simulink model "Wind_Turbine_Model"  (R2023a)
settings: Solver=VariableStepAuto  StartTime=0.0  StopTime=65  RelTol=1e-3
values from neighbouring files (symbols this model uses):
  Cbus = 80e-3*n_wt_agg*u^2    (= 1.33333333333)    [param.m]
  D = 1e-3    (= 0.001)    [param.m]
  f = 50    [param.m]
  Fs = Vs * sqrt(2/3)/(2*pi*f)    [param.m]
  fsw = 4e3    (= 4000)    [param.m]
  Idr_rated = sqrt(2)*Is    [param.m]
  J = 127*n_wt_agg    (= 19050)    [param.m]
  ki_id = (wni^2)*Lr*sigma    (= 3.27733001332)    [param.m]
  ki_idg = (wnig^2)*Lg    (= 0.263189450696)    [param.m]
  ki_iq = ki_id    (= 3.27733001332)    [param.m]
  ki_iqg = ki_idg    (= 0.263189450696)    [param.m]
  ki_v = -300000*n_wt_agg    (= -45000000)    [param.m]
  Kopt = ((0.5*rho*pi*(Radius^5)*Cp_max)/(lambda_opt^3))    (= 296454.198186)    [param.m]
  kp_id = (2*wni*sigma*Lr) - Rr    (= 0.00384733333333)    [param.m]
  kp_idg = ((2*wnig*Lg)-Rg)    (= 0.00167538274858)    [param.m]
  kp_iq = kp_id    (= 0.00384733333333)    [param.m]
  kp_iqg = kp_idg    (= 0.00167538274858)    [param.m]
  kp_v = -1000*n_wt_agg    (= -150000)    [param.m]
  Kpg = 1/(1.5*Vr*sqrt(2/3))    [param.m]
  Kqg = -Kpg    [param.m]
  lambda_opt = 7.2    [param.m]
  Lg = 400e-6 /n_wt_agg    (= 2.66666666667e-06)    [param.m]
  Lm = 2.5e-3 /n_wt_agg    (= 1.66666666667e-05)    [param.m]
  Lr = Lm + Lsi    (= 1.72466666667e-05)    [param.m]
  Ls = Lm + Lsi    (= 1.72466666667e-05)    [param.m]
  Lsi = 0.087e-3 /n_wt_agg    (= 5.8e-07)    [param.m]
  N = 100    [param.m]
  n_wt_agg = 150    [param.m]
  p = 2    [param.m]
  Ps = 2e6*n_wt_agg    (= 300000000)    [param.m]
  Radius = 42    [param.m]
  Rg = 20e-6 /n_wt_agg    (= 1.33333333333e-07)    [param.m]
  rho = 1.225    [param.m]
  Rr = 2.9e-3 /n_wt_agg    (= 1.93333333333e-05)    [param.m]
  Rs = 2.6e-3 /n_wt_agg    (= 1.73333333333e-05)    [param.m]
  sigma = 1 - Lm^2 / (Ls*Lr)    (= 0.0661284179513)    [param.m]
  smax = 1/3    (= 0.333333333333)    [param.m]
  tab_lambda = [0.1:0.01:11.8]    [param.m]
  Ts = 1/fsw/50    (= 5e-06)    [param.m]
  Vbus = 1150/u    (= 3450)    [param.m]
  Vs = 690    [param.m]
undefined symbols (not defined in the file or in its folder): Cp, DiscIntNeverNeededParam
libraries: spsSecondOrderFilterLib x10, simulink x5, spsThreePhaseVIMeasurementLib x4, spsPower3phInstantaneousLib x4, spsPiSectionLineLib x3, spsGroundLib x3, spsThreePhaseTransformerTwoWindingsLib x2, spsThreePhaseProgrammableVoltageSourceLib x2, spsUniversalBridgeLib x2, spsPWMGenerator2LevelLib x2, spsThreePhaseSeriesRLCBranchLib x2, spsAsynchronousMachineSIUnitsLib x1
(part 1 of 2)
settings Model: Creator=deleersnijde  LastModifiedBy=gdemuyter
settings DataIOCC: ReturnWorkspaceOutputs=off
settings RTWCC: GPUComputeCapability=5.0

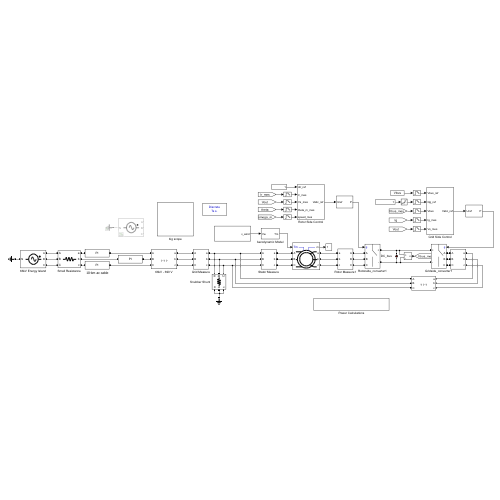
[thumbnail: Simulink's stored preview of the top-level diagram]
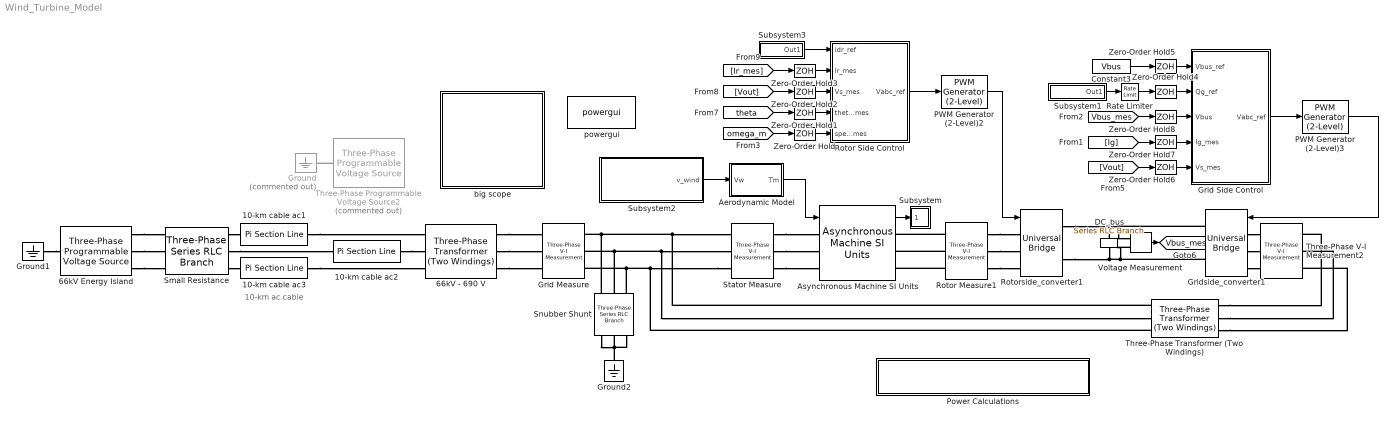
== system Wind_Turbine_Model ==
  note: 10-km ac cable
  10-km cable ac1 : spsPiSectionLineLib/Pi Section Line  LConnTagsString=__new0  RConnTagsString=__new0  Phases=1  PiSections=2  Length=10  Frequency=50  Resistance=0.034/(n_wt_agg/35)  Inductance=0.34e-3/(n_wt_agg/35)  Capacitance=0.29e-06*(n_wt_agg/35)  SpecifyConductance=off  Conductance=0  Measurements=None  Measurements2=None
  10-km cable ac2 : spsPiSectionLineLib/Pi Section Line  LConnTagsString=__new0  RConnTagsString=__new0  Phases=1  PiSections=2  Length=10  Frequency=50  Resistance=0.034/(n_wt_agg/35)  Inductance=0.34e-3/(n_wt_agg/35)  Capacitance=0.29e-06*(n_wt_agg/35)  SpecifyConductance=off  Conductance=0  Measurements=None  Measurements2=None
  10-km cable ac3 : spsPiSectionLineLib/Pi Section Line  LConnTagsString=__new0  RConnTagsString=__new0  Phases=1  PiSections=2  Length=10  Frequency=50  Resistance=0.034/(n_wt_agg/35)  Inductance=0.34e-3/(n_wt_agg/35)  Capacitance=0.29e-06*(n_wt_agg/35)  SpecifyConductance=off  Conductance=0  Measurements=None  Measurements2=None
  66kV - 690 V : spsThreePhaseTransformerTwoWindingsLib/Three-Phase Transformer (Two Windings)  Winding1Connection=Yg  Winding2Connection=Yg  CoreType=Three single-phase transformers  SetSaturation=off  Hysteresis=off  DataFile='hysteresis'  SetInitialFlux=off  Measurements=None  UNITS=pu  NominalPower=[ Ps , f ]  Winding1=[66000 0.025/100/25 0.015/25]  Winding2=[Vs 0.025/100/25 0.015/25]  Rm=500  Lm=500  L0=0.5  Saturation=[0 0;0.22957 0.012546;95.654 0.015891]  InitialFluxes=[ 0.8 , -0.8 , 0.7 ]  BreakLoop=off  DiscreteSolver=Trapezoidal iterative  DataType=off  TransfoNumber=1
  66kV Energy Island : spsThreePhaseProgrammableVoltageSourceLib/Three-Phase Programmable Voltage Source  PositiveSequence=[66e3 0 f]  VariationEntity=Amplitude  VariationType=Table of time-amplitude pairs  VariationTypeAlt=Step  VariationStep=0.5  VariationRate=10  VariationMagnitude=0.3  VariationFrequency=2  VariationTiming=[1 2]  VariationPhaseA=off  Amplitudes=[1 0.8 0.9 1.0]  TimeValues=[0 45 45.3 50]  HarmonicGeneration=off  HarmonicA=[3 0.2 -25 0]  HarmonicB=[2 0.15 35 2]  Timing="[0.05  3]"  BusType=swing  Pref=0  Qref=0  Qmin=-inf  Qmax=inf
  Aerodynamic Model : Subsystem
  Asynchronous Machine SI Units : spsAsynchronousMachineSIUnitsLib/Asynchronous Machine SI Units  RotorType=Wound  PresetModel=No  MechanicalLoad=Torque Tm  ShowDetailedParameters=on  ReferenceFrame=Rotor  Units=SI  MeasurementBus=off  NominalParameters=[Ps Vs f]  VoltageRatio=1/u  Stator=[Rs Lsi]  Rotor=[Rr Lsi]  Cage1=[0.4155 0.002066]  Cage2=[0.4168 0.0003495]  Lm=Lm  Mechanical=[J D 2]  PolePairs=2  InitialConditions=[0.454 0 0 0 0 0 0 0]  SimulateSaturation=off  Saturation=[14.03593122, 27.81365428, 53.79336849, 72.68890987, 97.98006896, 148.6815601, 215.7428561, 302.9841135, 428.7778367 ; 230, 322, 414, 460, 506, 552, 598, 644, 690]  LoadFlowParameters=1492000  TsPowergui=0  TsBlock=-1  IterativeModel=Trapezoidal non iterative  IterativeDiscreteModel=Trapezoidal non iterative  Pmec=1.492e+006
  Constant3 : Constant  Value=Vbus
  DC_bus : spsSeriesRLCBranchLib/Series RLC Branch  LConnTagsString=__new0  RConnTagsString=__new0  BranchType=C  Resistance=1  Inductance=1e-3  SetiL0=off  InitialCurrent=0  Capacitance=Cbus  Setx0=on  InitialVoltage=Vbus  Measurements=Branch voltage
  Grid Measure : spsThreePhaseVIMeasurementLib/Three-Phase V-I Measurement  VoltageMeasurement=phase-to-ground  SetLabelV=on  LabelV=Vout  Vpu=off  VpuLL=off  CurrentMeasurement=yes  SetLabelI=on  LabelI=Iout  Ipu=off  Pbase=100e6  Vbase=500e3  OutputType=Complex  PhasorSimulation=off  PSBequivalent=0
  Grid Side Control : Subsystem
  Gridside_converter1 : spsUniversalBridgeLib/Universal Bridge  Arms=3  SnubberResistance=5000  SnubberCapacitance=1e-6  Device=Ideal Switches  Ron=1e-3  Lon=0  ForwardVoltages="[  0  0  ]"  ForwardVoltage=0  GTOparameters=[ 10e-6 , 20e-6 ]  IGBTparameters=[ 1e-6 , 2e-6 ]  Measurements=UAB UBC UCA UDC voltages  Measurements_2=None  converterType=Rectifier
  Ground : spsGroundLib/Ground  Commented=on  LConnTagsString=a
  Ground1 : spsGroundLib/Ground  LConnTagsString=a
  Ground2 : spsGroundLib/Ground  LConnTagsString=a
  PWM Generator (2-Level)2 : spsPWMGenerator2LevelLib/PWM Generator (2-Level)  ModulatorType=Three-phase bridge (6 pulses)  ModulatorMode=Unsynchronized  Fc=fsw  Pc=0  nF=27  MinMax="[ -1  1 ]"  SamplingTechnique=Symmetrical regular (single edge)  ModulatingSignals=off  m=0.8  Freq=60  Phase=0  Ts=0  ShowCarrierOutport=off
  PWM Generator (2-Level)3 : spsPWMGenerator2LevelLib/PWM Generator (2-Level)  ModulatorType=Three-phase bridge (6 pulses)  ModulatorMode=Unsynchronized  Fc=fsw  Pc=0  nF=27  MinMax="[ -1  1 ]"  SamplingTechnique=Symmetrical regular (single edge)  ModulatingSignals=off  m=0.8  Freq=60  Phase=0  Ts=0  ShowCarrierOutport=off
  Power Calculations : Subsystem
  Rate Limiter : RateLimiter  RisingSlewLimit=Ps/4  FallingSlewLimit=-Ps/4  SampleTimeMode=inherited
  Rotor Measure1 : spsThreePhaseVIMeasurementLib/Three-Phase V-I Measurement  VoltageMeasurement=phase-to-ground  SetLabelV=on  LabelV=Vr_mes  Vpu=off  VpuLL=off  CurrentMeasurement=yes  SetLabelI=on  LabelI=Ir_mes  Ipu=off  Pbase=100e6  Vbase=500e3  OutputType=Complex  PhasorSimulation=off  PSBequivalent=0
  Rotor Side Control : Subsystem
  Rotorside_converter1 : spsUniversalBridgeLib/Universal Bridge  Arms=3  SnubberResistance=5000  SnubberCapacitance=1e-6  Device=Ideal Switches  Ron=1e-3  Lon=0  ForwardVoltages="[  0  0  ]"  ForwardVoltage=0  GTOparameters=[ 10e-6 , 20e-6 ]  IGBTparameters=[ 1e-6 , 2e-6 ]  Measurements=None  Measurements_2=None  converterType=Rectifier
  Small Resistance : spsThreePhaseSeriesRLCBranchLib/Three-Phase Series RLC Branch  LConnTagsString=A|B|C  RConnTagsString=A|B|C  BranchType=R  Resistance=0.01e-3  Inductance=0.01e-3  Capacitance=1e-6  Measurements=None
  Snubber Shunt : spsThreePhaseSeriesRLCBranchLib/Three-Phase Series RLC Branch  LConnTagsString=A|B|C  RConnTagsString=A|B|C  BranchType=R  Resistance=1e6  Inductance=Lg  Capacitance=1e-6  Measurements=None
  Stator Measure : spsThreePhaseVIMeasurementLib/Three-Phase V-I Measurement  VoltageMeasurement=phase-to-ground  SetLabelV=on  LabelV=Vs_mes_machine  Vpu=off  VpuLL=off  CurrentMeasurement=yes  SetLabelI=on  LabelI=Is_mes_machine  Ipu=off  Pbase=100e6  Vbase=500e3  OutputType=Complex  PhasorSimulation=off  PSBequivalent=0
  Subsystem : Subsystem
  Subsystem1 : Subsystem
  Subsystem2 : Subsystem
  Subsystem3 : Subsystem
  Three-Phase Programmable Voltage Source2 : spsThreePhaseProgrammableVoltageSourceLib/Three-Phase Programmable Voltage Source  Commented=on  PositiveSequence=[Vs 0 f]  VariationEntity=Amplitude  VariationType=Table of time-amplitude pairs  VariationTypeAlt=Step  VariationStep=0.5  VariationRate=10  VariationMagnitude=0.3  VariationFrequency=2  VariationTiming=[1 2]  VariationPhaseA=off  Amplitudes=[1 0.8 0.9 1.0]  TimeValues=[0 45 45.3 50]  HarmonicGeneration=off  HarmonicA=[3 0.2 -25 0]  HarmonicB=[2 0.15 35 2]  Timing="[0.05  3]"  BusType=swing  Pref=0  Qref=0  Qmin=-inf  Qmax=inf
  Three-Phase Transformer (Two Windings) : spsThreePhaseTransformerTwoWindingsLib/Three-Phase Transformer (Two Windings)  Winding1Connection=Yg  Winding2Connection=Yg  CoreType=Three single-phase transformers  SetSaturation=off  Hysteresis=off  DataFile='hysteresis'  SetInitialFlux=off  Measurements=None  UNITS=SI  NominalPower=[ Ps , f ]  Winding1=[690 0 0]  Winding2=[2070 Rg Lg]  Rm=500  Lm=500  L0=0.5  Saturation=[0 0;2840 2.152;1.1833e+06 2.7258]  InitialFluxes=[ 0.8 , -0.8 , 0.7 ]  BreakLoop=off  DiscreteSolver=Trapezoidal iterative  DataType=on  TransfoNumber=1
  Three-Phase V-I Measurement2 : spsThreePhaseVIMeasurementLib/Three-Phase V-I Measurement  VoltageMeasurement=phase-to-ground  SetLabelV=on  LabelV=Vg  Vpu=off  VpuLL=off  CurrentMeasurement=yes  SetLabelI=on  LabelI=Ig  Ipu=off  Pbase=100e6  Vbase=500e3  OutputType=Complex  PhasorSimulation=off  PSBequivalent=0
  Voltage Measurement : spsVoltageMeasurementLib/Voltage Measurement  PhasorSimulation=off  OutputType=Complex  PSBequivalent=0
  Zero-Order Hold{,1..8} (9 alike) : ZeroOrderHold  SampleTime=1/fsw
  big scope : Subsystem
  powergui : spspowerguiLib/powergui  Priority=1  SimulationMode=Discrete  SampleTime=Ts  frequency=60  Iterations=50  frequencyindice=50  Pbase=2e6  ErrMax=1e-4  UnitsV=kV  UnitsW=MW  buscounter=0  FunctionMessages=off  echomessages=off  EnableUseOfTLC=off  CurrentSourceSwitches=off  DisableSnubberDevices=off  DisableRonSwitches=off  DisableVfSwitches=off  DisplayEquations=off  AutomaticDiscreteSolvers=off  SolverType=Tustin/Backward Euler (TBE)  Interpol=off  ExternalGateDelay=off  methode=off  Ts=100  x0status=blocks  SPID=on  SwTol=0  HookPort=off  NonlinearTolerance=1e-4  nMaxIteration=100  ContinueOnMaxIteration=off  RestoreLinks=warning  ResistiveCurrentMeasurement=off  Frange=[0:2:500]  Ylog=off  Xlog=on  ShowGrid=off  save=off  variable=ZData  structure=0  ZoomFFT=off  StartTime=0.0  cycles=1  DisplayStyle=1  fundamental=60  FreqAxis=off  MaxFrequency=1000  frequencyindicesteady=1  RmsSteady=1  display=off
  tag scope: Vbus_mes=global
  wires:
  [Vout] -> Zero-Order Hold2/1
  Asynchronous Machine SI Units/1 -> Subsystem/1(In1)
  [theta] -> Zero-Order Hold1/1
  [omega_m] -> Zero-Order Hold/1
  Zero-Order Hold/1 -> Rotor Side Control/5(speed_mes)
  Zero-Order Hold1/1 -> Rotor Side Control/4(theta_m_mes)
  Zero-Order Hold2/1 -> Rotor Side Control/3(Vs_mes)
  Zero-Order Hold3/1 -> Rotor Side Control/2(Ir_mes)
  Aerodynamic Model/1(Tm) -> Asynchronous Machine SI Units/1
  Zero-Order Hold6/1 -> Grid Side Control/5(Vs_mes)
  [Vout] -> Zero-Order Hold6/1
  [Ig] -> Zero-Order Hold7/1
  Zero-Order Hold7/1 -> Grid Side Control/4(Ig_mes)
  Zero-Order Hold4/1 -> Grid Side Control/2(Qg_ref)
  Rate Limiter/1 -> Zero-Order Hold4/1
  Zero-Order Hold8/1 -> Grid Side Control/3(Vbus)
  [Vbus_mes] -> Zero-Order Hold8/1
  Grid Side Control/1(Vabc_ref) -> PWM Generator (2-Level)3/1
  Rotor Side Control/1(Vabc_ref) -> PWM Generator (2-Level)2/1
  Voltage Measurement/1 -> [Vbus_mes]
  Constant3/1 -> Zero-Order Hold5/1
  Zero-Order Hold5/1 -> Grid Side Control/1(Vbus_ref)
  Subsystem2/1(v_wind) -> Aerodynamic Model/1(Vw)
  [Ir_mes] -> Zero-Order Hold3/1
  Subsystem1/1(Out1) -> Rate Limiter/1
  Subsystem3/1(Out1) -> Rotor Side Control/1(idr_ref)
  PWM Generator (2-Level)3/1 -> Gridside_converter1/1
  PWM Generator (2-Level)2/1 -> Rotorside_converter1/1
  connections:
  Three-Phase Programmable Voltage Source2/LConn1 -- Ground/LConn1
  Three-Phase Transformer (Two Windings)/LConn1 -- Stator Measure/LConn1 -- Grid Measure/RConn1 -- Snubber Shunt/LConn1
  Stator Measure/LConn3 -- Three-Phase Transformer (Two Windings)/LConn3 -- Grid Measure/RConn3 -- Snubber Shunt/LConn3
  DC_bus/LConn1 -- Rotorside_converter1/RConn1 -- Gridside_converter1/RConn1 -- Voltage Measurement/LConn1
  DC_bus/RConn1 -- Rotorside_converter1/RConn2 -- Gridside_converter1/RConn2 -- Voltage Measurement/LConn2
  Gridside_converter1/LConn1 -- Three-Phase V-I Measurement2/LConn1
  Gridside_converter1/LConn2 -- Three-Phase V-I Measurement2/LConn2
  Gridside_converter1/LConn3 -- Three-Phase V-I Measurement2/LConn3
  Three-Phase Transformer (Two Windings)/RConn1 -- Three-Phase V-I Measurement2/RConn1
  Three-Phase Transformer (Two Windings)/RConn2 -- Three-Phase V-I Measurement2/RConn2
  Three-Phase Transformer (Two Windings)/RConn3 -- Three-Phase V-I Measurement2/RConn3
  Stator Measure/RConn1 -- Asynchronous Machine SI Units/LConn1
  Stator Measure/RConn2 -- Asynchronous Machine SI Units/LConn2
  Stator Measure/RConn3 -- Asynchronous Machine SI Units/LConn3
  Ground2/LConn1 -- Snubber Shunt/RConn3 -- Snubber Shunt/RConn1 -- Snubber Shunt/RConn2
  10-km cable ac2/RConn1 -- 66kV - 690 V/LConn2
  10-km cable ac1/RConn1 -- 66kV - 690 V/LConn1
  10-km cable ac3/RConn1 -- 66kV - 690 V/LConn3
  Three-Phase Transformer (Two Windings)/LConn2 -- Stator Measure/LConn2 -- Grid Measure/RConn2 -- Snubber Shunt/LConn2
  Ground1/LConn1 -- 66kV Energy Island/LConn1
  Small Resistance/RConn1 -- 10-km cable ac1/LConn1
  Small Resistance/RConn3 -- 10-km cable ac3/LConn1
  66kV Energy Island/RConn1 -- Small Resistance/LConn1
  66kV Energy Island/RConn2 -- Small Resistance/LConn2
  66kV Energy Island/RConn3 -- Small Resistance/LConn3
  Small Resistance/RConn2 -- 10-km cable ac2/LConn1
  66kV - 690 V/RConn1 -- Grid Measure/LConn1
  66kV - 690 V/RConn2 -- Grid Measure/LConn2
  66kV - 690 V/RConn3 -- Grid Measure/LConn3
  Rotor Measure1/RConn3 -- Asynchronous Machine SI Units/RConn3
  Rotor Measure1/RConn2 -- Asynchronous Machine SI Units/RConn2
  Rotor Measure1/LConn1 -- Rotorside_converter1/LConn1
  Rotor Measure1/LConn2 -- Rotorside_converter1/LConn2
  Rotor Measure1/LConn3 -- Rotorside_converter1/LConn3
  Rotor Measure1/RConn1 -- Asynchronous Machine SI Units/RConn1

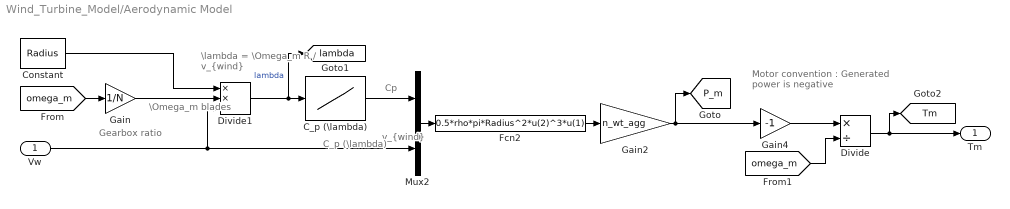
== system Wind_Turbine_Model/Aerodynamic Model ==
  note: v_{wind}
  note: C_p (\lambda)
  note: \lambda = \Omega_m R / v_{wind}
  note: Cp
  note: \Omega_m blades
  note: Motor convention : Generated power
      |  is negative
  note: Gearbox ratio
  Vw : Inport
  C_p (\lambda) : Lookup_n-D  NumberOfTableDimensions=1  BreakpointsForDimension1=tab_lambda  Table=Cp  InternalRulePriority=Speed  RndMeth=Simplest
  Constant : Constant  Value=Radius
  Divide : Product  Inputs=*/
  Divide1 : Product  Inputs=**/
  Fcn2 : Fcn  Expr=0.5*rho*pi*Radius^2*u(2)^3*u(1)
  Gain : Gain  Gain=1/N
  Gain2 : Gain  Gain=n_wt_agg
  Gain4 : Gain  Gain=-1
  Mux2 : Mux  Inputs=2
  Tm : Outport
  tag scope: P_m=global, Tm=global, lambda=global
  wires:
  [omega_m] -> Gain/1
  Gain/1 -> Divide1/2
  Vw/1 -> Divide1/3, Mux2/2
  Divide1/1 -> C_p (\lambda)/1, [lambda]  "lambda"
  C_p (\lambda)/1 -> Mux2/1
  Mux2/1 -> Fcn2/1
  Fcn2/1 -> Gain2/1
  Gain2/1 -> [P_m], Gain4/1
  [omega_m] -> Divide/2
  Divide/1 -> [Tm], Tm/1
  Constant/1 -> Divide1/1
  Gain4/1 -> Divide/1

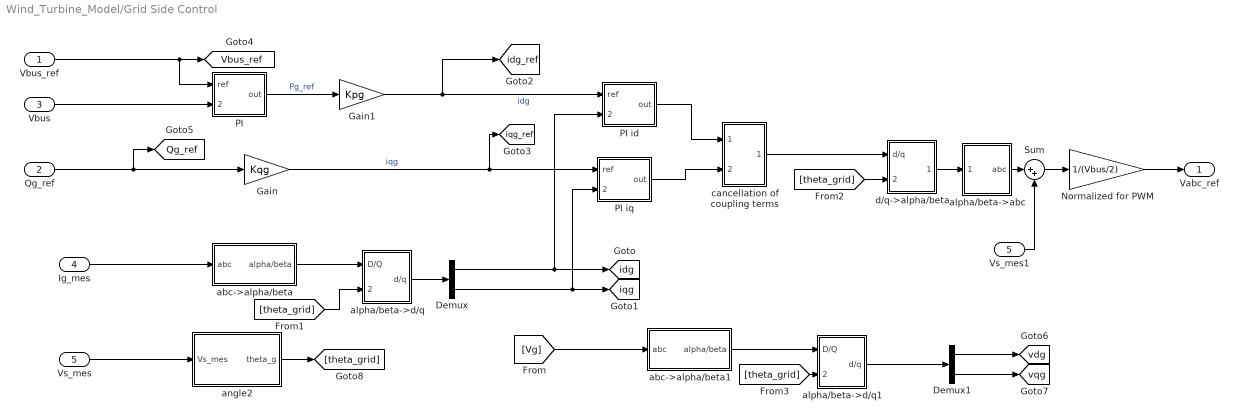
== system Wind_Turbine_Model/Grid Side Control ==
  Vbus_ref : Inport
  Qg_ref : Inport  Port=2
  Vbus : Inport  Port=3
  Ig_mes : Inport  Port=4
  Vs_mes : Inport  Port=5
  Demux : Demux  Outputs=2
  Demux1 : Demux  Outputs=2
  Gain : Gain  Gain=Kqg
  Gain1 : Gain  Gain=Kpg
  Normalized for PWM : Gain  Gain=1/(Vbus/2)
  "PI " : Subsystem
  PI id : Subsystem
  PI iq : Subsystem
  Sum : Sum  Inputs=|++
  Vs_mes1 : InportShadow  Port=5
  abc->alpha/beta : Subsystem
  abc->alpha/beta1 : Subsystem
  alpha/beta->abc : Subsystem
  alpha/beta->d/q : Subsystem
  alpha/beta->d/q1 : Subsystem
  angle2 : Subsystem
  cancellation of coupling terms : Subsystem
  d/q->alpha/beta : Subsystem
  Vabc_ref : Outport
  tag scope: Qg_ref=global, Vbus_ref=global, idg=global, idg_ref=global, iqg=global, iqg_ref=global, vdg=global, vqg=global
  wires:
  d/q->alpha/beta/1(D/Q) -> alpha/beta->abc/1(D/Q)
  Ig_mes/1 -> abc->alpha/beta/1(abc)
  abc->alpha/beta/1(alpha/beta) -> alpha/beta->d/q/1(D/Q)
  Normalized for PWM/1 -> Vabc_ref/1
  Vs_mes/1 -> angle2/1(Vs_mes)
  PI id/1(out) -> cancellation of coupling terms/1(Vd*)
  PI iq/1(out) -> cancellation of coupling terms/2(Vq*)
  alpha/beta->d/q/1(d/q) -> Demux/1
  Vbus_ref/1 -> [Vbus_ref], "PI "/1(ref)
  Gain/1 -> PI iq/1(ref), [iqg_ref]  "iqg"
  "PI "/1(out) -> Gain1/1  "Pg_ref"
  Gain1/1 -> [idg_ref], PI id/1(ref)  "idg"
  Qg_ref/1 -> [Qg_ref], Gain/1
  alpha/beta->abc/1(abc) -> Sum/1
  Sum/1 -> Normalized for PWM/1
  cancellation of coupling terms/1(out) -> d/q->alpha/beta/1(d/q)
  [Vg] -> abc->alpha/beta1/1(abc)
  abc->alpha/beta1/1(alpha/beta) -> alpha/beta->d/q1/1(D/Q)
  alpha/beta->d/q1/1(d/q) -> Demux1/1
  Demux1/2 -> [vqg]
  Demux1/1 -> [vdg]
  Vbus/1 -> "PI "/2(meas)
  Demux/1 -> [idg], PI id/2(meas)
  Demux/2 -> [iqg], PI iq/2(meas)
  [theta_grid] -> alpha/beta->d/q/2(theta)
  [theta_grid] -> d/q->alpha/beta/2(theta)
  [theta_grid] -> alpha/beta->d/q1/2(theta)
  angle2/1(theta_g) -> [theta_grid]
  Vs_mes1/1 -> Sum/2

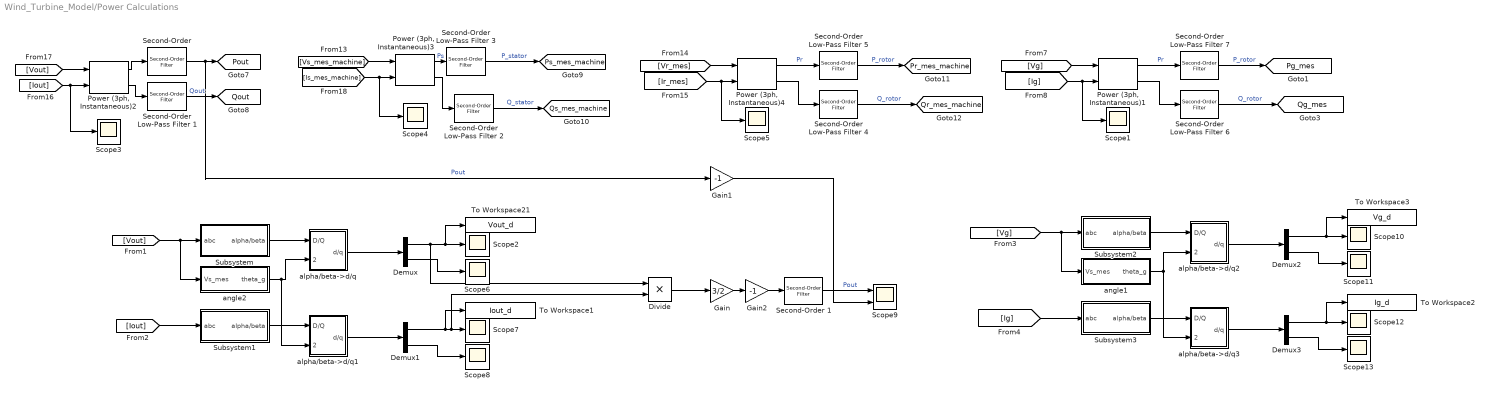
== system Wind_Turbine_Model/Power Calculations ==
  Demux{,1..3} (4 alike) : Demux  Outputs=2
  Divide : Product  Inputs=**
  Gain : Gain  Gain=3/2
  Gain1 : Gain  Gain=-1
  Gain2 : Gain  Gain=-1
  Power (3ph, Instantaneous){1..4} (4 alike) : spsPower3phInstantaneousLib/Power (3ph, Instantaneous)
  Scope{1..8,10..13} (12 alike) : Scope
  Scope9 : Scope  NumInputPorts=2
  "Second-Order " : spsSecondOrderFilterLib/Second-Order Filter  FilterType=Lowpass  Fo=17  Zeta=0.7  Ts=7.4074e-05  Initialize=off  Vac_Init="[0,  0,  60]"  Vdc_Init=0  PlotResponse=off  FreqRange=[0, 500, 1]
      settings: AttributesFormatString=f0=%<Fo>
  Second-Order 1 : spsSecondOrderFilterLib/Second-Order Filter  FilterType=Lowpass  Fo=17  Zeta=0.7  Ts=7.4074e-05  Initialize=off  Vac_Init="[0,  0,  60]"  Vdc_Init=0  PlotResponse=off  FreqRange=[0, 500, 1]
      settings: AttributesFormatString=f0=%<Fo>
  Second-Order Low-Pass Filter {1..7} (7 alike) : spsSecondOrderFilterLib/Second-Order Filter  FilterType=Lowpass  Fo=17  Zeta=0.7  Ts=7.4074e-05  Initialize=off  Vac_Init="[0,  0,  60]"  Vdc_Init=0  PlotResponse=off  FreqRange=[0, 500, 1]
      settings: AttributesFormatString=f0=%<Fo>
  Subsystem : Subsystem
  Subsystem1 : Subsystem
  Subsystem2 : Subsystem
  Subsystem3 : Subsystem
  To Workspace1 : ToWorkspace  VariableName=Iout_d  SaveFormat=Timeseries  SampleTime=-1
  To Workspace2 : ToWorkspace  VariableName=Ig_d  SaveFormat=Timeseries  SampleTime=-1
  To Workspace21 : ToWorkspace  VariableName=Vout_d  SaveFormat=Timeseries  SampleTime=-1
  To Workspace3 : ToWorkspace  VariableName=Vg_d  SaveFormat=Timeseries  SampleTime=-1
  alpha/beta->d/q : Subsystem
  alpha/beta->d/q1 : Subsystem
  alpha/beta->d/q2 : Subsystem
  alpha/beta->d/q3 : Subsystem
  angle1 : Subsystem
  angle2 : Subsystem
  tag scope: Pg_mes=global, Pout=global, Pr_mes_machine=global, Ps_mes_machine=global, Qg_mes=global, Qout=global, Qr_mes_machine=global, Qs_mes_machine=global
  wires:
  "Power (3ph, Instantaneous)2"/2 -> Second-Order Low-Pass Filter 1/1
  Second-Order Low-Pass Filter 1/1 -> [Qout]  "Qout"
  Second-Order Low-Pass Filter 3/1 -> [Ps_mes_machine]  "P_stator"
  "Power (3ph, Instantaneous)1"/2 -> Second-Order Low-Pass Filter 6/1
  [Iout] -> Scope3/1, "Power (3ph, Instantaneous)2"/2
  "Power (3ph, Instantaneous)4"/2 -> Second-Order Low-Pass Filter 4/1
  [Ig] -> "Power (3ph, Instantaneous)1"/2, Scope1/1
  "Power (3ph, Instantaneous)3"/1 -> Second-Order Low-Pass Filter 3/1  "Ps"
  Second-Order Low-Pass Filter 4/1 -> [Qr_mes_machine]  "Q_rotor"
  Second-Order Low-Pass Filter 6/1 -> [Qg_mes]  "Q_rotor"
  "Second-Order "/1 -> Gain1/1, [Pout]  "Pout"
  [Ir_mes] -> Scope5/1, "Power (3ph, Instantaneous)4"/2
  Second-Order Low-Pass Filter 7/1 -> [Pg_mes]  "P_rotor"
  [Is_mes_machine] -> Scope4/1, "Power (3ph, Instantaneous)3"/2
  Second-Order Low-Pass Filter 5/1 -> [Pr_mes_machine]  "P_rotor"
  "Power (3ph, Instantaneous)2"/1 -> "Second-Order "/1
  [Vs_mes_machine] -> "Power (3ph, Instantaneous)3"/1
  Second-Order Low-Pass Filter 2/1 -> [Qs_mes_machine]  "Q_stator"
  [Vg] -> "Power (3ph, Instantaneous)1"/1
  "Power (3ph, Instantaneous)3"/2 -> Second-Order Low-Pass Filter 2/1
  [Vout] -> "Power (3ph, Instantaneous)2"/1
  "Power (3ph, Instantaneous)4"/1 -> Second-Order Low-Pass Filter 5/1  "Pr"
  "Power (3ph, Instantaneous)1"/1 -> Second-Order Low-Pass Filter 7/1  "Pr"
  [Vr_mes] -> "Power (3ph, Instantaneous)4"/1
  [Vout] -> angle2/1(Vs_mes), Subsystem/1(abc)
  Subsystem/1(alpha/beta) -> alpha/beta->d/q/1(D/Q)
  alpha/beta->d/q/1(d/q) -> Demux/1
  Demux/1 -> Divide/1, To Workspace21/1, Scope2/1
  Demux/2 -> Scope6/1
  Demux1/2 -> Scope8/1
  Demux1/1 -> Divide/2, Scope7/1, To Workspace1/1
  alpha/beta->d/q1/1(d/q) -> Demux1/1
  Subsystem1/1(alpha/beta) -> alpha/beta->d/q1/1(D/Q)
  angle2/1(theta_g) -> alpha/beta->d/q1/2(theta), alpha/beta->d/q/2(theta)
  [Iout] -> Subsystem1/1(abc)
  Divide/1 -> Gain/1
  Second-Order 1/1 -> Scope9/1  "Pout"
  Gain1/1 -> Scope9/2
  Gain/1 -> Gain2/1
  Gain2/1 -> Second-Order 1/1
  [Ig] -> Subsystem3/1(abc)
  angle1/1(theta_g) -> alpha/beta->d/q2/2(theta), alpha/beta->d/q3/2(theta)
  Subsystem3/1(alpha/beta) -> alpha/beta->d/q3/1(D/Q)
  alpha/beta->d/q3/1(d/q) -> Demux3/1
  Demux3/1 -> To Workspace2/1, Scope12/1
  Demux3/2 -> Scope13/1
  Demux2/2 -> Scope11/1
  Demux2/1 -> Scope10/1, To Workspace3/1
  alpha/beta->d/q2/1(d/q) -> Demux2/1
  Subsystem2/1(alpha/beta) -> alpha/beta->d/q2/1(D/Q)
  [Vg] -> Subsystem2/1(abc), angle1/1(Vs_mes)

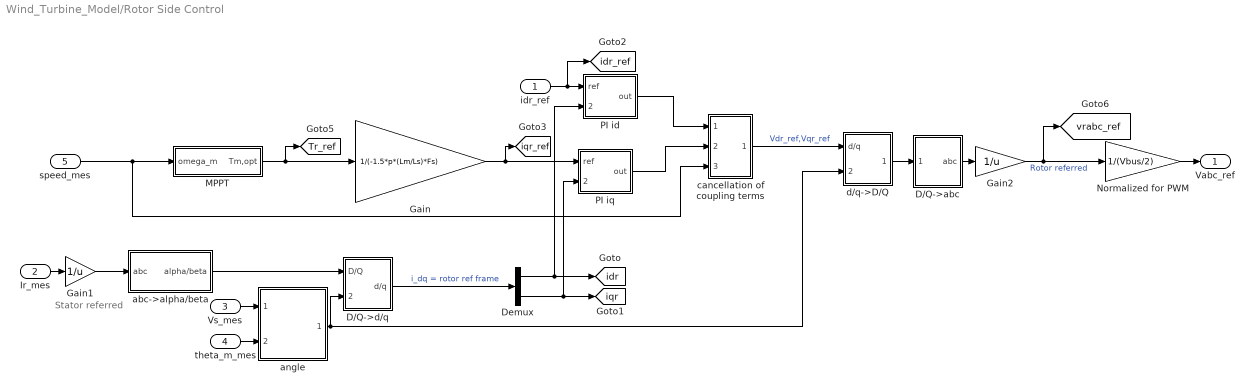
== system Wind_Turbine_Model/Rotor Side Control ==
  note: Stator referred
  idr_ref : Inport
  Ir_mes : Inport  Port=2
  Vs_mes : Inport  Port=3
  theta_m_mes : Inport  Port=4
  speed_mes : Inport  Port=5
  D/Q->abc : Subsystem
  D/Q->d/q : Subsystem
  Demux : Demux  Outputs=2
  Gain : Gain  Gain=1/(-1.5*p*(Lm/Ls)*Fs)
  Gain1 : Gain  Gain=1/u
  Gain2 : Gain  Gain=1/u
  MPPT : Subsystem
  Normalized for PWM : Gain  Gain=1/(Vbus/2)
  PI id : Subsystem
  PI iq : Subsystem
  abc->alpha/beta : Subsystem
  angle : Subsystem
  cancellation of coupling terms : Subsystem
  d/q->D/Q : Subsystem
  Vabc_ref : Outport
  tag scope: Tr_ref=global, idr=global, idr_ref=global, iqr=global, iqr_ref=global, vrabc_ref=global
  wires:
  Ir_mes/1 -> Gain1/1
  theta_m_mes/1 -> angle/2(theta_m)
  Vs_mes/1 -> angle/1(Vs_mes)
  angle/1(theta_r) -> d/q->D/Q/2(theta), D/Q->d/q/2(theta)
  PI id/1(out) -> cancellation of coupling terms/1(Vd*)
  PI iq/1(out) -> cancellation of coupling terms/2(Vq*)
  cancellation of coupling terms/1(out) -> d/q->D/Q/1(d/q)  "Vdr_ref,Vqr_ref"
  speed_mes/1 -> cancellation of coupling terms/3(omega_m), MPPT/1(omega_m)
  D/Q->d/q/1(d/q) -> Demux/1  "i_dq = rotor ref frame"
  Demux/1 -> PI id/2(meas), [idr]
  Demux/2 -> [iqr], PI iq/2(meas)
  Gain/1 -> [iqr_ref], PI iq/1(ref)
  idr_ref/1 -> [idr_ref], PI id/1(ref)
  Gain1/1 -> abc->alpha/beta/1(abc)
  Normalized for PWM/1 -> Vabc_ref/1
  D/Q->abc/1(abc) -> Gain2/1
  Gain2/1 -> Normalized for PWM/1, [vrabc_ref]  "Rotor referred"
  abc->alpha/beta/1(alpha/beta) -> D/Q->d/q/1(D/Q)
  d/q->D/Q/1(D/Q) -> D/Q->abc/1(D/Q)
  MPPT/1(Tm,opt) -> [Tr_ref], Gain/1

== system Wind_Turbine_Model/Subsystem ==
  In1 : Inport
  Bus Selector : BusSelector  OutputSignals=Mechanical.Rotor angle thetam (rad),Mechanical.Rotor speed (wm),Mechanical.Electromagnetic torque Te (N*m)
  Second-Order Low-Pass Filter 3 : spsSecondOrderFilterLib/Second-Order Filter  FilterType=Lowpass  Fo=17  Zeta=0.7  Ts=7.4074e-05  Initialize=off  Vac_Init="[0,  0,  60]"  Vdc_Init=0  PlotResponse=off  FreqRange=[0, 500, 1]
      settings: AttributesFormatString=f0=%<Fo>
  tag scope: Tr=global, omega_m=global, theta=global
  wires:
  Bus Selector/2 -> Second-Order Low-Pass Filter 3/1  "<Rotor speed (wm)>"
  In1/1 -> Bus Selector/1
  Bus Selector/1 -> [theta]  "<Rotor angle thetam (rad)>"
  Bus Selector/3 -> [Tr]  "<Electromagnetic torque Te (N*m)>"
  Second-Order Low-Pass Filter 3/1 -> [omega_m]

== system Wind_Turbine_Model/Subsystem1 ==
  Constant4 : Constant  Value=0
  Step : Step  Time=30  After=-0.2*Ps  SampleTime=0
  Sum14 : Sum  Inputs=++|
  Out1 : Outport
  wires:
  Constant4/1 -> Sum14/2
  Step/1 -> Sum14/1
  Sum14/1 -> Out1/1

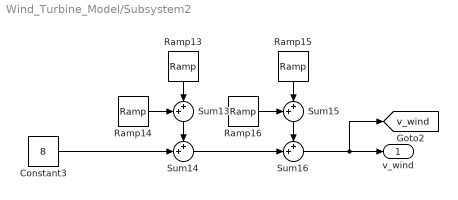
== system Wind_Turbine_Model/Subsystem2 ==
  Constant3 : Constant  Value=8
  Ramp13 : simulink/Sources/Ramp  slope=-1  start=18  InitialOutput=0
  Ramp14 : simulink/Sources/Ramp  slope=1  start=17  InitialOutput=0
  Ramp15 : simulink/Sources/Ramp  slope=-1  start=36  InitialOutput=0
  Ramp16 : simulink/Sources/Ramp  slope=1  start=35  InitialOutput=0
  Sum{13..16} (4 alike) : Sum  Inputs=++|
  v_wind : Outport
  tag scope: v_wind=global
  wires:
  Sum16/1 -> [v_wind], v_wind/1
  Ramp14/1 -> Sum13/1
  Ramp13/1 -> Sum13/2
  Sum13/1 -> Sum14/1
  Sum15/1 -> Sum16/1
  Ramp15/1 -> Sum15/2
  Ramp16/1 -> Sum15/1
  Sum14/1 -> Sum16/2
  Constant3/1 -> Sum14/2

== system Wind_Turbine_Model/Subsystem3 ==
  Constant4 : Constant  Value=0
  Step : Step  Time=55  After=Idr_rated*0.2  SampleTime=0
  Sum14 : Sum  Inputs=++|
  Out1 : Outport
  wires:
  Step/1 -> Sum14/1
  Constant4/1 -> Sum14/2
  Sum14/1 -> Out1/1

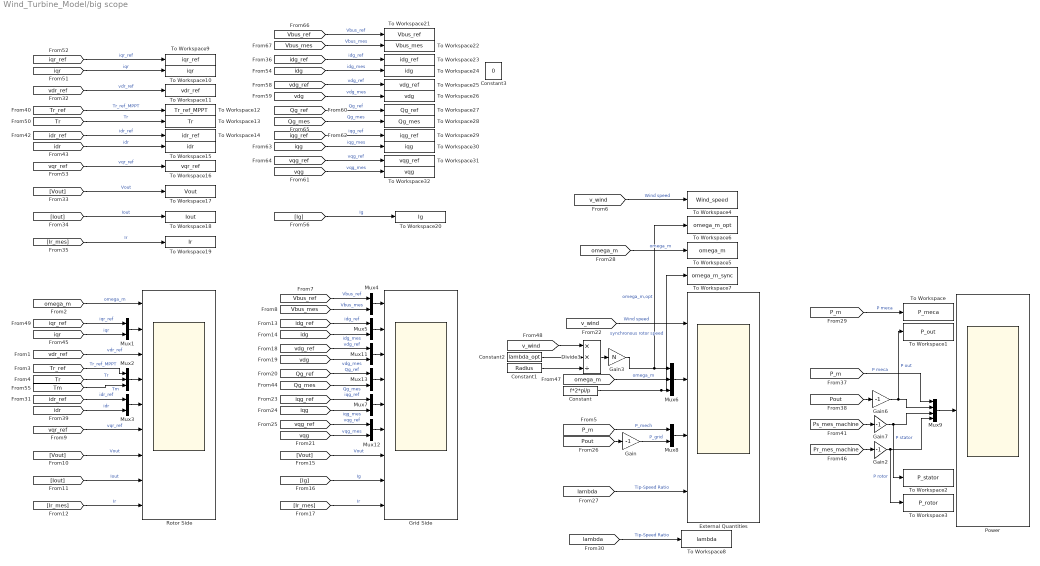
== system Wind_Turbine_Model/big scope ==
  Constant : Constant  Value=f*2*pi/p
  Constant1 : Constant  Value=Radius
  Constant2 : Constant  Value=lambda_opt
  Constant3 : Constant  Value=0
  Divide3 : Product  Inputs=**/
  External Quantities : Scope  NumInputPorts=4
  Gain{,2,6..7} (4 alike) : Gain  Gain=-1
  Gain3 : Gain  Gain=N
  Grid Side : Scope  NumInputPorts=9
  Mux{1,3..5,7..8,11..13} (9 alike) : Mux  Inputs=2
  Mux2 : Mux  Inputs=3
  Mux6 : Mux  Inputs=3
  Mux9 : Mux
  Power : Scope
  Rotor Side : Scope  NumInputPorts=9
  To Workspace : ToWorkspace  VariableName=P_meca  SaveFormat=Timeseries  SampleTime=-1
  To Workspace1 : ToWorkspace  VariableName=P_out  SaveFormat=Timeseries  SampleTime=-1
  To Workspace10 : ToWorkspace  VariableName=iqr  SaveFormat=Timeseries  SampleTime=-1
  To Workspace11 : ToWorkspace  VariableName=vdr_ref  SaveFormat=Timeseries  SampleTime=-1
  To Workspace12 : ToWorkspace  VariableName=Tr_ref_MPPT  SaveFormat=Timeseries  SampleTime=-1
  To Workspace13 : ToWorkspace  VariableName=Tr  SaveFormat=Timeseries  SampleTime=-1
  To Workspace14 : ToWorkspace  VariableName=idr_ref  SaveFormat=Timeseries  SampleTime=-1
  To Workspace15 : ToWorkspace  VariableName=idr  SaveFormat=Timeseries  SampleTime=-1
  To Workspace16 : ToWorkspace  VariableName=vqr_ref  SaveFormat=Timeseries  SampleTime=-1
  To Workspace17 : ToWorkspace  VariableName=Vout  SaveFormat=Timeseries  SampleTime=-1
  To Workspace18 : ToWorkspace  VariableName=Iout  SaveFormat=Timeseries  SampleTime=-1
  To Workspace19 : ToWorkspace  VariableName=Ir  SaveFormat=Timeseries  SampleTime=-1
  To Workspace2 : ToWorkspace  VariableName=P_stator  SaveFormat=Timeseries  SampleTime=-1
  To Workspace20 : ToWorkspace  VariableName=Ig  SaveFormat=Timeseries  SampleTime=-1
  To Workspace21 : ToWorkspace  VariableName=Vbus_ref  SaveFormat=Timeseries  SampleTime=-1
  To Workspace22 : ToWorkspace  VariableName=Vbus_mes  SaveFormat=Timeseries  SampleTime=-1
  To Workspace23 : ToWorkspace  VariableName=idg_ref  SaveFormat=Timeseries  SampleTime=-1
  To Workspace24 : ToWorkspace  VariableName=idg  SaveFormat=Timeseries  SampleTime=-1
  To Workspace25 : ToWorkspace  VariableName=vdg_ref  SaveFormat=Timeseries  SampleTime=-1
  To Workspace26 : ToWorkspace  VariableName=vdg  SaveFormat=Timeseries  SampleTime=-1
  To Workspace27 : ToWorkspace  VariableName=Qg_ref  SaveFormat=Timeseries  SampleTime=-1
  To Workspace28 : ToWorkspace  VariableName=Qg_mes  SaveFormat=Timeseries  SampleTime=-1
  To Workspace29 : ToWorkspace  VariableName=iqg_ref  SaveFormat=Timeseries  SampleTime=-1
  To Workspace3 : ToWorkspace  VariableName=P_rotor  SaveFormat=Timeseries  SampleTime=-1
  To Workspace30 : ToWorkspace  VariableName=iqg  SaveFormat=Timeseries  SampleTime=-1
  To Workspace31 : ToWorkspace  VariableName=vqg_ref  SaveFormat=Timeseries  SampleTime=-1
  To Workspace32 : ToWorkspace  VariableName=vqg  SaveFormat=Timeseries  SampleTime=-1
  To Workspace4 : ToWorkspace  VariableName=Wind_speed  SaveFormat=Timeseries  SampleTime=-1
  To Workspace5 : ToWorkspace  VariableName=omega_m  SaveFormat=Timeseries  SampleTime=-1
  To Workspace6 : ToWorkspace  VariableName=omega_m_opt  SaveFormat=Timeseries  SampleTime=-1
  To Workspace7 : ToWorkspace  VariableName=omega_m_sync  SaveFormat=Timeseries  SampleTime=-1
  To Workspace8 : ToWorkspace  VariableName=lambda  SaveFormat=Timeseries  SampleTime=-1
  To Workspace9 : ToWorkspace  VariableName=iqr_ref  SaveFormat=Timeseries  SampleTime=-1
  wires:
  [iqr] -> Mux1/2  "iqr"
  Mux1/1 -> Rotor Side/2
  [Tr_ref] -> Mux2/1  "Tr_ref_MPPT"
  Mux2/1 -> Rotor Side/4
  Mux3/1 -> Rotor Side/5
  [idr_ref] -> Mux3/1  "idr_ref"
  [vqr_ref] -> Rotor Side/6  "vqr_ref"
  [Vout] -> Rotor Side/7  "Vout"
  [Iout] -> Rotor Side/8  "Iout"
  [Ir_mes] -> Rotor Side/9  "Ir"
  [Ig] -> Grid Side/8  "Ig"
  [iqg_ref] -> Mux7/1  "iqg_ref"
  [Vout] -> Grid Side/7  "Vout"
  [Ir_mes] -> Grid Side/9  "Ir"
  [iqg] -> Mux7/2  "iqg_mes"
  [Vbus_ref] -> Mux4/1  "Vbus_ref"
  Mux7/1 -> Grid Side/5
  [Vbus_mes] -> Mux4/2  "Vbus_mes"
  Mux5/1 -> Grid Side/2
  [idg] -> Mux5/2  "idg_mes"
  Mux4/1 -> Grid Side/1
  [idg_ref] -> Mux5/1  "idg_ref"
  [omega_m] -> Rotor Side/1  "omega_m"
  Gain/1 -> Mux8/2  "P_grid"
  [Pout] -> Gain/1
  Mux8/1 -> External Quantities/3
  Mux6/1 -> External Quantities/2
  [v_wind] -> External Quantities/1  "Wind speed"
  [omega_m] -> Mux6/2  "omega_m"
  Constant/1 -> To Workspace7/1, Mux6/3  "synchronous rotor speed"
  [P_m] -> Mux8/1  "P_mech"
  [vdg_ref] -> Mux11/1  "vdg_ref"
  [vdg] -> Mux11/2  "vdg_mes"
  Mux11/1 -> Grid Side/3
  Gain6/1 -> To Workspace1/1, Mux9/2  "P out"
  [Ps_mes_machine] -> Gain7/1
  Gain7/1 -> To Workspace2/1, Mux9/3  "P stator"
  [Pr_mes_machine] -> Gain2/1
  [P_m] -> Mux9/1  "P meca"
  Mux9/1 -> Power/1
  [Pout] -> Gain6/1
  Gain2/1 -> To Workspace3/1, Mux9/4  "P rotor"
  [vqg] -> Mux12/2  "vqg_mes"
  [vqg_ref] -> Mux12/1  "vqg_ref"
  Mux12/1 -> Grid Side/6
  [Qg_ref] -> Mux13/1  "Qg_ref"
  [Qg_mes] -> Mux13/2  "Qg_mes"
  Mux13/1 -> Grid Side/4
  [iqr_ref] -> Mux1/1  "iqr_ref"
  [vdr_ref] -> Rotor Side/3  "vdr_ref"
  [Tr] -> Mux2/2  "Tr"
  [idr] -> Mux3/2  "idr"
  [v_wind] -> Divide3/1
  Constant2/1 -> Divide3/2
  Constant1/1 -> Divide3/3
  Divide3/1 -> Gain3/1
  Gain3/1 -> To Workspace6/1, Mux6/1  "omega_m,opt"
  [lambda] -> External Quantities/4  "Tip-Speed Ratio"
  [v_wind] -> To Workspace4/1  "Wind speed"
  [omega_m] -> To Workspace5/1  "omega_m"
  [P_m] -> To Workspace/1  "P meca"
  [lambda] -> To Workspace8/1  "Tip-Speed Ratio"
  [iqr_ref] -> To Workspace9/1  "iqr_ref"
  [iqr] -> To Workspace10/1  "iqr"
  [vdr_ref] -> To Workspace11/1  "vdr_ref"
  [Tr_ref] -> To Workspace12/1  "Tr_ref_MPPT"
  [Tr] -> To Workspace13/1  "Tr"
  [idr_ref] -> To Workspace14/1  "idr_ref"
  [idr] -> To Workspace15/1  "idr"
  [vqr_ref] -> To Workspace16/1  "vqr_ref"
  [Vout] -> To Workspace17/1  "Vout"
  [Iout] -> To Workspace18/1  "Iout"
  [Ir_mes] -> To Workspace19/1  "Ir"
  [Ig] -> To Workspace20/1  "Ig"
  [Vbus_ref] -> To Workspace21/1  "Vbus_ref"
  [Vbus_mes] -> To Workspace22/1  "Vbus_mes"
  [idg_ref] -> To Workspace23/1  "idg_ref"
  [idg] -> To Workspace24/1  "idg_mes"
  [vdg_ref] -> To Workspace25/1  "vdg_ref"
  [Qg_ref] -> To Workspace27/1  "Qg_ref"
  [vdg] -> To Workspace26/1  "vdg_mes"
  [Qg_mes] -> To Workspace28/1  "Qg_mes"
  [iqg_ref] -> To Workspace29/1  "iqg_ref"
  [iqg] -> To Workspace30/1  "iqg_mes"
  [vqg_ref] -> To Workspace31/1  "vqg_ref"
  [vqg] -> To Workspace32/1  "vqg_mes"
  [Tm] -> Mux2/3  "Tm"

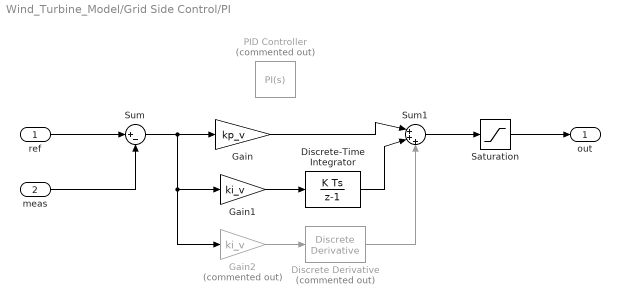
== system Wind_Turbine_Model/Grid Side Control/PI  ==
  ref : Inport
  meas : Inport  Port=2
  Discrete Derivative : simulink/Discrete/Discrete Derivative  Commented=on  gainval=1.0  ICPrevScaledInput=0.0  OutMin=[-Ps*smax]  OutMax=[Ps*smax]  OutDataType=fixdt(1, 16)  OutScaling=2^-10  DoSatur=off
  Discrete-Time Integrator : DiscreteIntegrator  SampleTime=1/fsw  LimitOutput=on  UpperSaturationLimit=Ps*smax  LowerSaturationLimit=-Ps*smax  ICPrevOutput=DiscIntNeverNeededParam  ICPrevScaledInput=DiscIntNeverNeededParam
  Gain : Gain  Gain=kp_v
  Gain1 : Gain  Gain=ki_v
  Gain2 : Gain  Commented=on  Gain=ki_v
  PID Controller : slpidlib/PID Controller  Commented=on  Controller=PI  Form=Parallel  TimeDomain=Continuous-time  UseExternalTs=off  SampleTime=-1  IntegratorMethod=Forward Euler  FilterMethod=Forward Euler  ControllerParametersSource=internal  P=kp_v  I=ki_v  UseKiTs=off  D=0  N=100  UseFilter=on  TunerSelectOption=Transfer Function Based (PID Tuner App)  InitialConditionSource=internal  InitialConditionForIntegrator=0  InitialConditionForFilter=0  DifferentiatorICPrevScaledInput=0  ExternalReset=none  TrackingMode=off  Kt=1  LimitOutput=on  SatLimitsSource=internal  UpperSaturationLimit=Ps*smax  LowerSaturationLimit=-Ps*smax  LinearizeAsGain=on  AntiWindupMode=clamping  Kb=1  LimitIntegrator=on  UpperIntegratorSaturationLimit=Ps*smax  LowerIntegratorSaturationLimit=-Ps*smax  POutMin=[]  POutMax=[]  IOutMin=[]  IOutMax=[]  DOutMin=[]  DOutMax=[]  NOutMin=[]  NOutMax=[]  SumOutMin=[]  SumOutMax=[]  SaturationOutMin=[]  SaturationOutMax=[]  PParamMin=[]  PParamMax=[]  IParamMin=[]  IParamMax=[]  DParamMin=[]  DParamMax=[]  NParamMin=[]  NParamMax=[]  KbParamMin=[]  KbParamMax=[]  KtParamMin=[]  KtParamMax=[]  KbOutMin=[]  KbOutMax=[]  KtOutMin=[]  KtOutMax=[]  IntegratorOutMin=[]  IntegratorOutMax=[]  FilterOutMin=[]  FilterOutMax=[]  SumI1OutMin=[]  SumI1OutMax=[]  SumI2OutMin=[]  SumI2OutMax=[]  SumI3OutMin=[]  SumI3OutMax=[]  SumI4OutMin=[]  SumI4OutMax=[]  SumDOutMin=[]  SumDOutMax=[]  DifferentiatorOutMin=[]  DifferentiatorOutMax=[]  FilterDiffOutCoefMin=[]  FilterDiffOutCoefMax=[]  ReciprocalOutMin=[]  ReciprocalOutMax=[]  SumDenOutMin=[]  SumDenOutMax=[]  SumNumOutMin=[]  SumNumOutMax=[]  DivideOutMin=[]  DivideOutMax=[]  UdiffTsProdOutMin=[]  UdiffTsProdOutMax=[]  NTsProdOutMin=[]  NTsProdOutMax=[]  UintegralTsProdOutMin=[]  UintegralTsProdOutMax=[]  UngainTsProdOutMin=[]  UngainTsProdOutMax=[]  ClampingZeroOutDataTypeStr=Inherit: Inherit via back propagation  ClampingZeroOutMin=[]  ClampingZeroOutMax=[]  FilterDenConstantOutDataTypeStr=Inherit: Inherit via back propagation  FilterDenConstantOutMin=[]  FilterDenConstantOutMax=[]  PCopyOutDataTypeStr=Inherit: Inherit via back propagation  PCopyOutMin=[]  PCopyOutMax=[]  NCopyOutDataTypeStr=Inherit: Inherit via back propagation  NCopyOutMin=[]  NCopyOutMax=[]  IntegratorContinuousStateAttributes=''  IntegratorStateMustResolveToSignalObject=off  IntegratorRTWStateStorageClass=Auto  FilterContinuousStateAttributes=''  FilterStateMustResolveToSignalObject=off  FilterRTWStateStorageClass=Auto  ParallelPVariant=InternalParameters  IdealPVariant=Disabled  IVariant=InternalParameters  DVariant=Disabled  IntegratorVariant=Continuous  SatVariant=Enabled  AWVariant=ContClampingParallel  PCopyVariant=Disabled  TRVariant=Disabled  FdbkBlocksVariant=Forward  IdealPFdbkVariant=Disabled  SatFdbkVariant=Disabled  DerivativeFilterVariant=Disabled  NVariant=Disabled  NCopyVariant=Disabled_SignalSpec  FilterICVariant=Disabled  IntegratorICVariant=InternalICs  ExternalResetVariant=Disabled  TRSumVariant=Passthrough  SumFdbkVariant=Disabled  SumVariant=Sum_PI  TsampFilterVariant=InternalTs  TsampNgainVariant=Passthrough  TsampIntegralVariant=Disabled_SignalSpec  ExternalSaturationOutDataTypeStr=Inherit: Same as second input
  Saturation : Saturate  UpperLimit=Ps*smax  LowerLimit=-Ps*smax
  Sum : Sum  Inputs=|+-
  Sum1 : Sum  Inputs=|+++
  out : Outport
  wires:
  Saturation/1 -> out/1
  ref/1 -> Sum/1
  meas/1 -> Sum/2
  Sum/1 -> Gain2/1, Gain1/1, Gain/1
  Gain/1 -> Sum1/1
  Gain1/1 -> Discrete-Time Integrator/1
  Discrete-Time Integrator/1 -> Sum1/2
  Sum1/1 -> Saturation/1
  Gain2/1 -> Discrete Derivative/1
  Discrete Derivative/1 -> Sum1/3

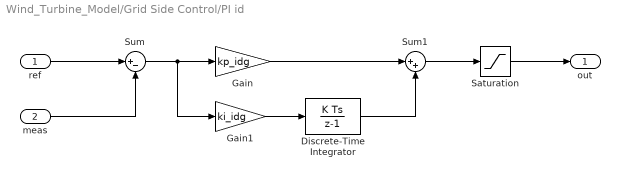
== system Wind_Turbine_Model/Grid Side Control/PI id ==
  ref : Inport
  meas : Inport  Port=2
  Discrete-Time Integrator : DiscreteIntegrator  SampleTime=1/fsw  LimitOutput=on  UpperSaturationLimit=Vbus/sqrt(3)  LowerSaturationLimit=-Vbus/sqrt(3)  ICPrevOutput=DiscIntNeverNeededParam  ICPrevScaledInput=DiscIntNeverNeededParam
  Gain : Gain  Gain=kp_idg
  Gain1 : Gain  Gain=ki_idg
  Saturation : Saturate  UpperLimit=Vbus/sqrt(3)  LowerLimit=-Vbus/sqrt(3)
  Sum : Sum  Inputs=|+-
  Sum1 : Sum  Inputs=|++
  out : Outport
  wires:
  Saturation/1 -> out/1
  ref/1 -> Sum/1
  meas/1 -> Sum/2
  Sum/1 -> Gain1/1, Gain/1
  Gain/1 -> Sum1/1
  Gain1/1 -> Discrete-Time Integrator/1
  Discrete-Time Integrator/1 -> Sum1/2
  Sum1/1 -> Saturation/1

== system Wind_Turbine_Model/Grid Side Control/PI iq ==
  ref : Inport
  meas : Inport  Port=2
  Discrete-Time Integrator : DiscreteIntegrator  SampleTime=1/fsw  LimitOutput=on  UpperSaturationLimit=Vbus/sqrt(3)  LowerSaturationLimit=-Vbus/sqrt(3)  ICPrevOutput=DiscIntNeverNeededParam  ICPrevScaledInput=DiscIntNeverNeededParam
  Gain : Gain  Gain=kp_iqg
  Gain1 : Gain  Gain=ki_iqg
  Saturation : Saturate  UpperLimit=Vbus/sqrt(3)  LowerLimit=-Vbus/sqrt(3)
  Sum : Sum  Inputs=|+-
  Sum1 : Sum  Inputs=|++
  out : Outport
  wires:
  Saturation/1 -> out/1
  ref/1 -> Sum/1
  meas/1 -> Sum/2
  Sum/1 -> Gain1/1, Gain/1
  Gain/1 -> Sum1/1
  Gain1/1 -> Discrete-Time Integrator/1
  Discrete-Time Integrator/1 -> Sum1/2
  Sum1/1 -> Saturation/1

== system Wind_Turbine_Model/Grid Side Control/abc->alpha//beta ==
  abc : Inport
  Fcn1 : Fcn  Expr=2/3 * (u[1]-u[2]/2-u[3]/2)
  Fcn2 : Fcn  Expr=2/3 * (u[2] * (sqrt(3)/2) - u[3]*(sqrt(3)/2))
  Mux : Mux  Inputs=2
  alpha/beta : Outport
  wires:
  Fcn2/1 -> Mux/2
  Fcn1/1 -> Mux/1
  Mux/1 -> alpha/beta/1
  abc/1 -> Fcn1/1, Fcn2/1

== system Wind_Turbine_Model/Grid Side Control/abc->alpha//beta1 ==
  abc : Inport
  Fcn1 : Fcn  Expr=2/3 * (u[1]-u[2]/2-u[3]/2)
  Fcn2 : Fcn  Expr=2/3 * (u[2] * (sqrt(3)/2) - u[3]*(sqrt(3)/2))
  Mux : Mux  Inputs=2
  alpha/beta : Outport
  wires:
  Fcn2/1 -> Mux/2
  Fcn1/1 -> Mux/1
  Mux/1 -> alpha/beta/1
  abc/1 -> Fcn1/1, Fcn2/1

== system Wind_Turbine_Model/Grid Side Control/alpha//beta->abc ==
  note: D/Q = alpha/beta en fait
  D/Q : Inport
  Fcn : Fcn  Expr=u[1]
  Fcn1 : Fcn  Expr=-(u[1]/2) + u[2]*(sqrt(3)/2)
  Fcn2 : Fcn  Expr=-(u[1]/2) - u[2]*(sqrt(3)/2)
  Mux : Mux  Inputs=3
  abc : Outport
  wires:
  D/Q/1 -> Fcn2/1, Fcn1/1, Fcn/1
  Fcn1/1 -> Mux/2
  Mux/1 -> abc/1
  Fcn2/1 -> Mux/3
  Fcn/1 -> Mux/1

== system Wind_Turbine_Model/Grid Side Control/alpha//beta->d//q ==
  D/Q : Inport
  theta : Inport  Port=2
  Fcn : Fcn  Expr=u[1]*cos(u[3]) + u[2]*sin(u[3])
  Fcn1 : Fcn  Expr=-u[1]*sin(u[3]) + u[2]*cos(u[3])
  Mux : Mux  Inputs=2
  Mux1 : Mux  Inputs=2
  d/q : Outport
  wires:
  Mux/1 -> d/q/1
  D/Q/1 -> Mux1/1
  theta/1 -> Mux1/2
  Fcn/1 -> Mux/1
  Mux1/1 -> Fcn/1, Fcn1/1
  Fcn1/1 -> Mux/2

== system Wind_Turbine_Model/Grid Side Control/alpha//beta->d//q1 ==
  D/Q : Inport
  theta : Inport  Port=2
  Fcn : Fcn  Expr=u[1]*cos(u[3]) + u[2]*sin(u[3])
  Fcn1 : Fcn  Expr=-u[1]*sin(u[3]) + u[2]*cos(u[3])
  Mux : Mux  Inputs=2
  Mux1 : Mux  Inputs=2
  d/q : Outport
  wires:
  Fcn1/1 -> Mux/2
  Mux1/1 -> Fcn1/1, Fcn/1
  Fcn/1 -> Mux/1
  theta/1 -> Mux1/2
  D/Q/1 -> Mux1/1
  Mux/1 -> d/q/1

== system Wind_Turbine_Model/Grid Side Control/angle2 ==
  Vs_mes : Inport
  Demux : Demux  Outputs=2
  Simple PLL : Trigonometry  Operator=atan2
  abc->alpha/beta : Subsystem
  theta_g : Outport
  wires:
  Vs_mes/1 -> abc->alpha/beta/1(abc)
  abc->alpha/beta/1(alpha/beta) -> Demux/1
  Demux/1 -> Simple PLL/2
  Demux/2 -> Simple PLL/1
  Simple PLL/1 -> theta_g/1  "theta_g"

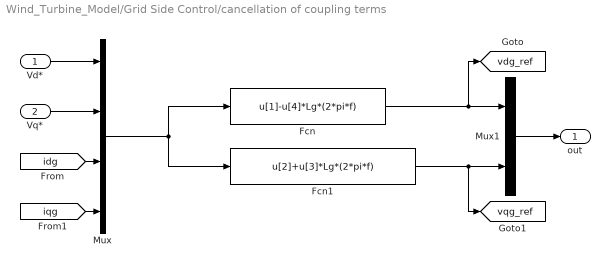
== system Wind_Turbine_Model/Grid Side Control/cancellation of coupling terms ==
  Vd* : Inport
  Vq* : Inport  Port=2
  Fcn : Fcn  Expr=u[1]-u[4]*Lg*(2*pi*f)
  Fcn1 : Fcn  Expr=u[2]+u[3]*Lg*(2*pi*f)
  Mux : Mux
  Mux1 : Mux  Inputs=2
  out : Outport
  tag scope: vdg_ref=global, vqg_ref=global
  wires:
  Vd*/1 -> Mux/1
  Vq*/1 -> Mux/2
  [idg] -> Mux/3
  [iqg] -> Mux/4
  Mux/1 -> Fcn/1, Fcn1/1
  Mux1/1 -> out/1
  Fcn/1 -> [vdg_ref], Mux1/1
  Fcn1/1 -> [vqg_ref], Mux1/2

== system Wind_Turbine_Model/Grid Side Control/d//q->alpha//beta ==
  d/q : Inport
  theta : Inport  Port=2
  Fcn : Fcn  Expr=u[1]*cos(u[3])-u[2]*sin(u[3])
  Fcn1 : Fcn  Expr=u[1]*sin(u[3])+u[2]*cos(u[3])
  Mux : Mux  Inputs=2
  Mux1 : Mux  Inputs=2
  D/Q : Outport
  wires:
  Mux/1 -> D/Q/1
  d/q/1 -> Mux1/1
  theta/1 -> Mux1/2
  Fcn/1 -> Mux/1
  Mux1/1 -> Fcn/1, Fcn1/1
  Fcn1/1 -> Mux/2

== system Wind_Turbine_Model/Power Calculations/Subsystem ==
  abc : Inport
  Fcn1 : Fcn  Expr=2/3 * (u[1]-u[2]/2-u[3]/2)
  Fcn2 : Fcn  Expr=2/3 * (u[2] * (sqrt(3)/2) - u[3]*(sqrt(3)/2))
  Mux : Mux  Inputs=2
  alpha/beta : Outport
  wires:
  Fcn2/1 -> Mux/2
  abc/1 -> Fcn1/1, Fcn2/1
  Fcn1/1 -> Mux/1
  Mux/1 -> alpha/beta/1

== system Wind_Turbine_Model/Power Calculations/Subsystem1 ==
  abc : Inport
  Fcn1 : Fcn  Expr=2/3 * (u[1]-u[2]/2-u[3]/2)
  Fcn2 : Fcn  Expr=2/3 * (u[2] * (sqrt(3)/2) - u[3]*(sqrt(3)/2))
  Mux : Mux  Inputs=2
  alpha/beta : Outport
  wires:
  Mux/1 -> alpha/beta/1
  Fcn1/1 -> Mux/1
  abc/1 -> Fcn2/1, Fcn1/1
  Fcn2/1 -> Mux/2

== system Wind_Turbine_Model/Power Calculations/Subsystem2 ==
  abc : Inport
  Fcn1 : Fcn  Expr=2/3 * (u[1]-u[2]/2-u[3]/2)
  Fcn2 : Fcn  Expr=2/3 * (u[2] * (sqrt(3)/2) - u[3]*(sqrt(3)/2))
  Mux : Mux  Inputs=2
  alpha/beta : Outport
  wires:
  Mux/1 -> alpha/beta/1
  Fcn1/1 -> Mux/1
  abc/1 -> Fcn2/1, Fcn1/1
  Fcn2/1 -> Mux/2

== system Wind_Turbine_Model/Power Calculations/Subsystem3 ==
  abc : Inport
  Fcn1 : Fcn  Expr=2/3 * (u[1]-u[2]/2-u[3]/2)
  Fcn2 : Fcn  Expr=2/3 * (u[2] * (sqrt(3)/2) - u[3]*(sqrt(3)/2))
  Mux : Mux  Inputs=2
  alpha/beta : Outport
  wires:
  Fcn2/1 -> Mux/2
  abc/1 -> Fcn1/1, Fcn2/1
  Fcn1/1 -> Mux/1
  Mux/1 -> alpha/beta/1

== system Wind_Turbine_Model/Power Calculations/alpha//beta->d//q ==
  D/Q : Inport
  theta : Inport  Port=2
  Fcn : Fcn  Expr=u[1]*cos(u[3]) + u[2]*sin(u[3])
  Fcn1 : Fcn  Expr=-u[1]*sin(u[3]) + u[2]*cos(u[3])
  Mux : Mux  Inputs=2
  Mux1 : Mux  Inputs=2
  d/q : Outport
  wires:
  Mux/1 -> d/q/1
  D/Q/1 -> Mux1/1
  theta/1 -> Mux1/2
  Fcn/1 -> Mux/1
  Mux1/1 -> Fcn/1, Fcn1/1
  Fcn1/1 -> Mux/2

== system Wind_Turbine_Model/Power Calculations/alpha//beta->d//q1 ==
  D/Q : Inport
  theta : Inport  Port=2
  Fcn : Fcn  Expr=u[1]*cos(u[3]) + u[2]*sin(u[3])
  Fcn1 : Fcn  Expr=-u[1]*sin(u[3]) + u[2]*cos(u[3])
  Mux : Mux  Inputs=2
  Mux1 : Mux  Inputs=2
  d/q : Outport
  wires:
  Fcn1/1 -> Mux/2
  Mux1/1 -> Fcn1/1, Fcn/1
  Fcn/1 -> Mux/1
  theta/1 -> Mux1/2
  D/Q/1 -> Mux1/1
  Mux/1 -> d/q/1

== system Wind_Turbine_Model/Power Calculations/alpha//beta->d//q2 ==
  D/Q : Inport
  theta : Inport  Port=2
  Fcn : Fcn  Expr=u[1]*cos(u[3]) + u[2]*sin(u[3])
  Fcn1 : Fcn  Expr=-u[1]*sin(u[3]) + u[2]*cos(u[3])
  Mux : Mux  Inputs=2
  Mux1 : Mux  Inputs=2
  d/q : Outport
  wires:
  Fcn1/1 -> Mux/2
  Mux1/1 -> Fcn1/1, Fcn/1
  Fcn/1 -> Mux/1
  theta/1 -> Mux1/2
  D/Q/1 -> Mux1/1
  Mux/1 -> d/q/1

== system Wind_Turbine_Model/Power Calculations/alpha//beta->d//q3 ==
  D/Q : Inport
  theta : Inport  Port=2
  Fcn : Fcn  Expr=u[1]*cos(u[3]) + u[2]*sin(u[3])
  Fcn1 : Fcn  Expr=-u[1]*sin(u[3]) + u[2]*cos(u[3])
  Mux : Mux  Inputs=2
  Mux1 : Mux  Inputs=2
  d/q : Outport
  wires:
  Mux/1 -> d/q/1
  D/Q/1 -> Mux1/1
  theta/1 -> Mux1/2
  Fcn/1 -> Mux/1
  Mux1/1 -> Fcn/1, Fcn1/1
  Fcn1/1 -> Mux/2

== system Wind_Turbine_Model/Power Calculations/angle1 ==
  Vs_mes : Inport
  Demux : Demux  Outputs=2
  Simple PLL : Trigonometry  Operator=atan2
  abc->alpha/beta : Subsystem
  theta_g : Outport
  wires:
  Simple PLL/1 -> theta_g/1  "theta_g"
  Demux/2 -> Simple PLL/1
  Demux/1 -> Simple PLL/2
  abc->alpha/beta/1(alpha/beta) -> Demux/1
  Vs_mes/1 -> abc->alpha/beta/1(abc)

== system Wind_Turbine_Model/Power Calculations/angle2 ==
  Vs_mes : Inport
  Demux : Demux  Outputs=2
  Simple PLL : Trigonometry  Operator=atan2
  abc->alpha/beta : Subsystem
  theta_g : Outport
  wires:
  Vs_mes/1 -> abc->alpha/beta/1(abc)
  abc->alpha/beta/1(alpha/beta) -> Demux/1
  Demux/1 -> Simple PLL/2
  Demux/2 -> Simple PLL/1
  Simple PLL/1 -> theta_g/1  "theta_g"

== system Wind_Turbine_Model/Rotor Side Control/D//Q->abc ==
  note: D/Q = alpha/beta en fait
  D/Q : Inport
  Fcn : Fcn  Expr=u[1]
  Fcn1 : Fcn  Expr=-(u[1]/2) + u[2]*(sqrt(3)/2)
  Fcn2 : Fcn  Expr=-(u[1]/2) - u[2]*(sqrt(3)/2)
  Mux : Mux  Inputs=3
  abc : Outport
  wires:
  D/Q/1 -> Fcn2/1, Fcn1/1, Fcn/1
  Fcn1/1 -> Mux/2
  Mux/1 -> abc/1
  Fcn2/1 -> Mux/3
  Fcn/1 -> Mux/1

== system Wind_Turbine_Model/Rotor Side Control/D//Q->d//q ==
  D/Q : Inport
  theta : Inport  Port=2
  Fcn : Fcn  Expr=u[1]*cos(u[3]) + u[2]*sin(u[3])
  Fcn1 : Fcn  Expr=-u[1]*sin(u[3]) + u[2]*cos(u[3])
  Mux : Mux  Inputs=2
  Mux1 : Mux  Inputs=2
  d/q : Outport
  wires:
  Mux/1 -> d/q/1
  D/Q/1 -> Mux1/1
  theta/1 -> Mux1/2
  Fcn/1 -> Mux/1
  Mux1/1 -> Fcn/1, Fcn1/1
  Fcn1/1 -> Mux/2

== system Wind_Turbine_Model/Rotor Side Control/MPPT ==
  note: \omega_m
  note: \Omega_m
  note: \Omega^2_m
  note: T_{m,opt}
  omega_m : Inport
  Gain : Gain  Gain=1/N
  Gain1 : Gain  Gain=-Kopt
  Gain2 : Gain  Gain=1/N
  Gain3 : Gain  Gain=n_wt_agg
  Square : Math  Operator=square
  Tm,opt : Outport
  wires:
  omega_m/1 -> Gain/1
  Gain/1 -> Square/1
  Square/1 -> Gain1/1
  Gain1/1 -> Gain2/1
  Gain2/1 -> Gain3/1
  Gain3/1 -> Tm,opt/1

== system Wind_Turbine_Model/Rotor Side Control/PI id ==
  ref : Inport
  meas : Inport  Port=2
  Discrete-Time Integrator : DiscreteIntegrator  SampleTime=1/fsw  LimitOutput=on  UpperSaturationLimit=Vbus/sqrt(3)  LowerSaturationLimit=-Vbus/sqrt(3)  ICPrevOutput=DiscIntNeverNeededParam  ICPrevScaledInput=DiscIntNeverNeededParam
  Gain : Gain  Gain=kp_id
  Gain1 : Gain  Gain=ki_id
  Saturation : Saturate  UpperLimit=Vbus/sqrt(3)  LowerLimit=-Vbus/sqrt(3)
  Sum : Sum  Inputs=|+-
  Sum1 : Sum  Inputs=|++
  out : Outport
  wires:
  Saturation/1 -> out/1
  ref/1 -> Sum/1
  meas/1 -> Sum/2
  Sum/1 -> Gain1/1, Gain/1
  Gain/1 -> Sum1/1
  Gain1/1 -> Discrete-Time Integrator/1
  Discrete-Time Integrator/1 -> Sum1/2
  Sum1/1 -> Saturation/1

== system Wind_Turbine_Model/Rotor Side Control/PI iq ==
  ref : Inport
  meas : Inport  Port=2
  Discrete-Time Integrator : DiscreteIntegrator  SampleTime=1/fsw  LimitOutput=on  UpperSaturationLimit=Vbus/sqrt(3)  LowerSaturationLimit=-Vbus/sqrt(3)  ICPrevOutput=DiscIntNeverNeededParam  ICPrevScaledInput=DiscIntNeverNeededParam
  Gain : Gain  Gain=kp_iq
  Gain1 : Gain  Gain=ki_iq
  Saturation : Saturate  UpperLimit=Vbus/sqrt(3)  LowerLimit=-Vbus/sqrt(3)
  Sum : Sum  Inputs=|+-
  Sum1 : Sum  Inputs=|++
  out : Outport
  wires:
  Saturation/1 -> out/1
  ref/1 -> Sum/1
  meas/1 -> Sum/2
  Sum/1 -> Gain1/1, Gain/1
  Gain/1 -> Sum1/1
  Gain1/1 -> Discrete-Time Integrator/1
  Discrete-Time Integrator/1 -> Sum1/2
  Sum1/1 -> Saturation/1

== system Wind_Turbine_Model/Rotor Side Control/abc->alpha//beta ==
  abc : Inport
  Fcn1 : Fcn  Expr=2/3 * (u[1]-u[2]/2-u[3]/2)
  Fcn2 : Fcn  Expr=2/3 * (u[2] * (sqrt(3)/2) - u[3]*(sqrt(3)/2))
  Mux : Mux  Inputs=2
  alpha/beta : Outport
  wires:
  Fcn2/1 -> Mux/2
  Fcn1/1 -> Mux/1
  Mux/1 -> alpha/beta/1
  abc/1 -> Fcn1/1, Fcn2/1

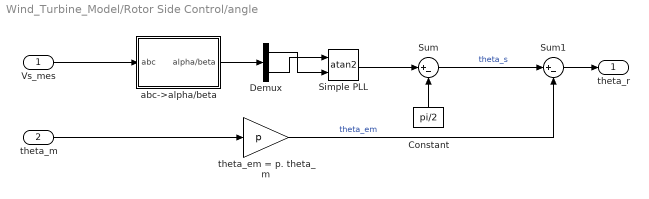
== system Wind_Turbine_Model/Rotor Side Control/angle ==
  Vs_mes : Inport
  theta_m : Inport  Port=2
  Constant : Constant  Value=pi/2
  Demux : Demux  Outputs=2
  Simple PLL : Trigonometry  Operator=atan2
  Sum : Sum  Inputs=|+-
  Sum1 : Sum  Inputs=|+-
  abc->alpha/beta : Subsystem
  theta_em = p. theta_m : Gain  Gain=p
  theta_r : Outport
  wires:
  Sum1/1 -> theta_r/1
  Vs_mes/1 -> abc->alpha/beta/1(abc)
  abc->alpha/beta/1(alpha/beta) -> Demux/1
  Demux/1 -> Simple PLL/2
  Demux/2 -> Simple PLL/1
  Simple PLL/1 -> Sum/1
  Sum/1 -> Sum1/1  "theta_s"
  theta_m/1 -> theta_em = p. theta_m/1
  theta_em = p. theta_m/1 -> Sum1/2  "theta_em"
  Constant/1 -> Sum/2
